simulink model "Geo_ma_T_v3"  (R2023b)
settings: Solver=VariableStepAuto  StartTime=0.0  StopTime=1  FixedStep=1e-3  MaxStep=1e-5  MinStep=0.00000000000001  RelTol=1e-5  AbsTol=1e-6
undefined symbols (not defined in the file): qi
settings Model: Creator=netoa  LastModifiedBy=neto
settings DebuggingCC: UnderSpecifiedDimensionMsg=error

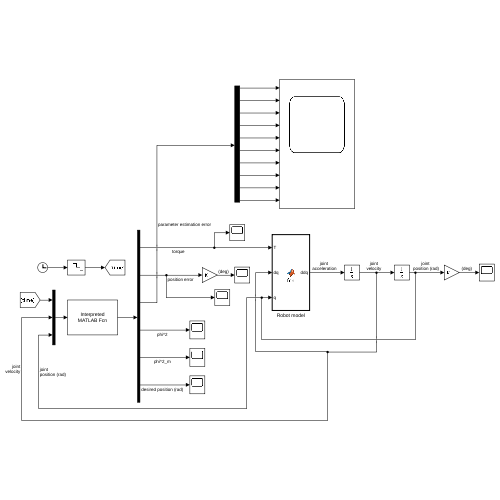
[thumbnail: Simulink's stored preview of the top-level diagram]
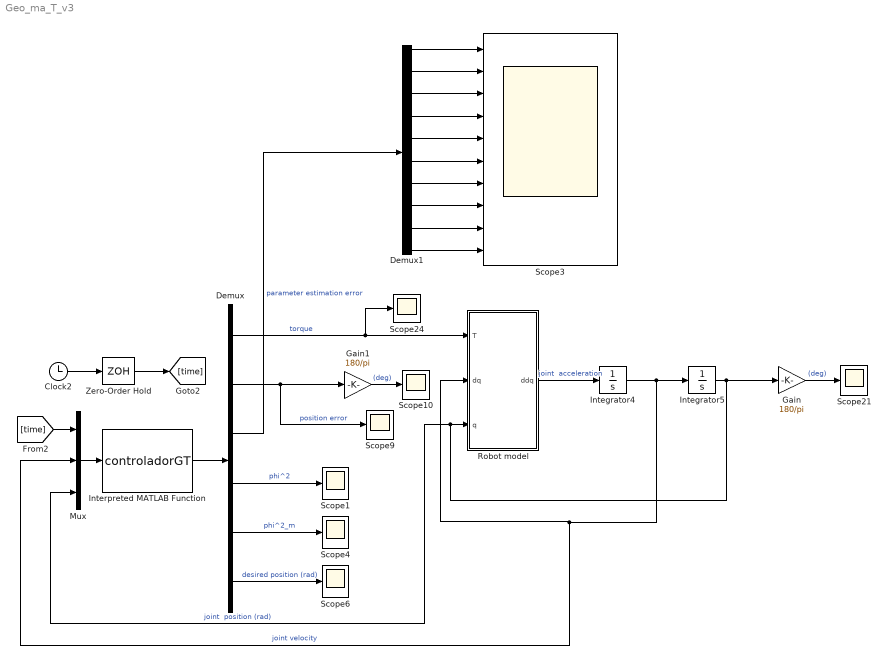
== system Geo_ma_T_v3 ==
  Clock2 : Clock
  Demux : Demux  Outputs=[3,3,10, 1, 1, 3]
  Demux1 : Demux  Outputs=10
  Gain : Gain  Gain=180/pi
  Gain1 : Gain  Gain=180/pi
  Integrator4 : Integrator  InitialCondition=[0; 0; 0]
  Integrator5 : Integrator  InitialCondition=qi
  Interpreted MATLAB Function : MATLABFcn  MATLABFcn=controladorGT  OutputDimensions=21
  Mux : Mux  Inputs=3
  Robot model : MATLAB Function  TreatAsAtomicUnit=on
  Scope{1,4,6,9..10,21,24} (7 alike) : Scope
  Scope3 : Scope  NumInputPorts=10
  Zero-Order Hold : ZeroOrderHold  SampleTime=-1
  wires:
  Integrator4/1 -> Integrator5/1, Robot model/2(dq), Mux/2  "joint velocity"
  Integrator5/1 -> Gain/1, Mux/3, Robot model/3(q)  "joint  position (rad)"
  Robot model/1(ddq) -> Integrator4/1  "joint  acceleration"
  Mux/1 -> Interpreted MATLAB Function/1
  [time] -> Mux/1
  Interpreted MATLAB Function/1 -> Demux/1
  Demux/1 -> Scope24/1, Robot model/1(T)  "torque"
  Demux/2 -> Gain1/1, Scope9/1  "position error"
  Clock2/1 -> Zero-Order Hold/1
  Zero-Order Hold/1 -> [time]
  Demux/4 -> Scope1/1  "phi^2"
  Demux1/7 -> Scope3/7
  Demux1/6 -> Scope3/6
  Demux1/8 -> Scope3/8
  Demux1/2 -> Scope3/2
  Demux1/5 -> Scope3/5
  Demux1/3 -> Scope3/3
  Demux1/4 -> Scope3/4
  Demux1/1 -> Scope3/1
  Demux/3 -> Demux1/1  "parameter estimation error"
  Demux/5 -> Scope4/1  "phi^2_m"
  Demux1/9 -> Scope3/9
  Demux1/10 -> Scope3/10
  Demux/6 -> Scope6/1  "desired position (rad)"
  Gain/1 -> Scope21/1  "(deg)"
  Gain1/1 -> Scope10/1  "(deg)"

== matlab function Geo_ma_T_v3/Robot model ==
  data: ddq output; T input; dq input; q input
function ddq    = fcn(T, dq, q)

g0 = 9.81; %gravity

% First derivative of the generalized coordinate (joint angular velocity)
dq1=dq(1);
dq2=dq(2);
dq3=dq(3);

% generalized coordinate (joint angular position)
q1=q(1);
q2=q(2);
q3=q(3);

% Robot +  payload parameters
vpi1 = 0.00349359;
vpi2 = 0.00248272;
vpi3 = 0.00459359;
vpi4 = 0.00006993;
vpi5 = 0.00465868;
vpi6 = 0.00076823;
vpi7 = 0.03526735;
vpi8 = 0.00744473;
vpi9 = 0.02191225;
vpi10 = 0.01712223;

%trigonometric expressions

s2=sin(q2);
s3=sin(q3);
s23=sin(q2+q3);
c2=cos(q2);
c3=cos(q3);
c23=cos(q2+q3);


%Inertia matrix H(q)

h11 = c2 * c2 * vpi1 + 2 * c2 * c23 * vpi2 + c23 * c23 * vpi3 + s23 * s23 * vpi4;
h12 = 0; h13 = 0; h21 = 0;
h22 = vpi1 + 2 * c3 * vpi2 + vpi5;
h23= c3 * vpi2 + vpi5;
h31 = 0;
h32 = c3 * vpi2 + vpi5;
h33 = vpi5;

H=[h11 h12 h13; h21 h22 h23; h31 h32 h33];

%Matrix C(q,\dot{q})

ce11 = -c2 * s2 * dq2 * vpi1 - 0.5 * (c2 * s23 * (dq2 + dq3) + s2 * c23 * dq2) * vpi2 - c23 * s23 * (dq2 + dq3) * vpi3 + c23 * s23 * (dq2 + dq3) * vpi4;
ce12 = -c2 * s2 * dq1 * vpi1 - 0.5 * (s2 * c23 + c2 * s23) * dq1 * vpi2 - s23 * c23 * dq1 * vpi3 + s23 * c23 * dq1 * vpi4;
ce13 = -0.5 * c2 * s23 * dq1 * vpi2 - c23 * s23 * dq1 * vpi3 + c23 * s23 * dq1 * vpi4;
ce21 = c2 * s2 * dq1 * vpi1 + 0.5 * (s2 * c23 + c2 * s23) * dq1 * vpi2 + s23 * c23 * dq1 * vpi3 - s23 * c23 * dq1 * vpi4;%%%
ce22 = -s3 * dq3 * vpi2;
ce23 = -s3 * (dq2 + dq3) * vpi2;
ce31 = 0.5 * c2 * s23 * dq1 * vpi2 + c23 * s23 * dq1 * vpi3 - c23 * s23 * dq1 * vpi4;
ce32 = s3 * dq2 * vpi2;
ce33 = 0.0;

C=[ce11 ce12 ce13; ce21 ce22 ce23; ce31 ce32 ce33];

%Matrix of joint viscous friction coeffcients D

d1=vpi6*dq1;
d2=vpi7*dq2;
d3=vpi8*dq3;

D=[d1; d2; d3];

%Gravity torque vector g(q)

g1 = 0;
g2 = g0 * (c2 * vpi9 + c23 * vpi10);
g3 = g0 * c23 * vpi10;

g=[g1; g2; g3];

%Output
ddq=(H^(-1))*(T-C*dq-D-g);
